simulink model "StateFlow_5"  (R2018a)
settings: Solver=FixedStepDiscrete  StartTime=0.0  StopTime=10.0  FixedStep=0.01  RelTol=1e-3
settings Model: SnapshotBufferSize=1000  Creator=Choaib ELMADI  LastModifiedBy=Choaib ELMADI

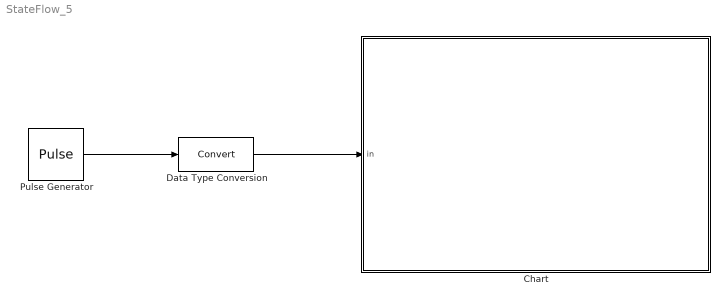
== system StateFlow_5 ==
  Chart : Stateflow chart  TreatAsAtomicUnit=on
  Data Type Conversion : DataTypeConversion
  Pulse Generator : DiscretePulseGenerator  PulseType=Time based  Period=0.1  PulseWidth=50
  wires:
  Data Type Conversion/1 -> Chart/1(in)
  Pulse Generator/1 -> Data Type Conversion/1

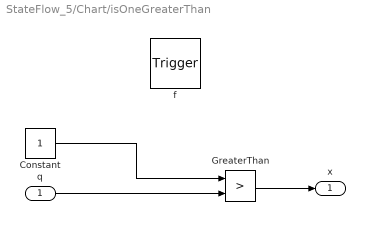
== system StateFlow_5/Chart/isOneGreaterThan ==
  q : Inport  OutDataTypeStr=double  PortDimensions=1
  f : TriggerPort  TriggerType=function-call  VariantControl=(inherit)
      settings: CopyFcn=Stateflow.SLINSF.SimulinkMan.removeBlockPreDeleteFcn  PreDeleteFcn=Stateflow.SLINSF.SimulinkMan.unsafePredeleteFcn
  Constant : Constant
  GreaterThan : RelationalOperator  Operator=>  OutDataTypeStr=boolean  RndMeth=Simplest
  x : Outport  OutDataTypeStr=boolean
  wires:
  GreaterThan/1 -> x/1
  q/1 -> GreaterThan/2
  Constant/1 -> GreaterThan/1

== stateflow chart StateFlow_5/Chart ==
  state f = factorial(q) [function]
    (default) -> (junction 26) : % Calculate Factorial
    (junction 26) -> (junction 27) : {i = 1; f = 1;}
    (junction 27) -> (junction 25) [order 1] : [i <= q]
    (junction 25) -> (junction 28) : {f = f * i;}
    (junction 28) -> (junction 27) : {i = i + 1;}
    (junction 27) -> (junction 29) [order 2]
  state x = isOneGreaterThan(q) [function]
  state ON_STATE
    en:
    var = mySqrt(9);
    fact = factorial(3);
  state OFF_STATE
    var = mySqrt(16);
    fact = factorial(4);
  (default) -> ON_STATE
  ON_STATE -> OFF_STATE : [isOneGreaterThan(in)]
  OFF_STATE -> ON_STATE : [~isOneGreaterThan(in)]
  data: q function_input; x function_output; q function_input; f function_output; q function_input double size=1; x function_output boolean; in input boolean; var local double; fact local double
  function x = mySqrt(q):
    | function x = mySqrt(q)
    |     x = sqrt(q);
    | end
